simulink model "gm_uz_pmsm_model_6ph_dq"  (R2023a)
settings: Solver=FixedStepAuto  StartTime=0.0  StopTime=0.8  RelTol=1e-3
undefined symbols (not defined in the file or in its folder): c, friction_coefficient, inertia, k_i_d, k_i_q, k_p_d, k_p_q, Kpd, L_d, L_q, L_x, L_y, L_z1, L_z2, polepair, psi_pm, R_1, static_friction_torque, Tnd
libraries: hdlmdlgenlib x51, slpidlib x2, pid_lib x1, spsdq0toAlphaBetaZeroLib x1
(part 2 of 2)

== system gm_uz_pmsm_model_6ph_dq/uz_pmsm_model_6ph_dq/Data Type Conversion14 ==
  In1 : Inport
  Data Type Conversion14 : DataTypeConversion  OutDataTypeStr=single  RndMeth=Nearest  SampleTime=1e-08  SaturateOnIntegerOverflow=off
  Data Type Conversion14_pd1 : Delay  DelayLength=3
  Out1 : Outport
  wires:
  In1/1 -> Data Type Conversion14/1
  Data Type Conversion14/1 -> Data Type Conversion14_pd1/1
  Data Type Conversion14_pd1/1 -> Out1/1

== system gm_uz_pmsm_model_6ph_dq/uz_pmsm_model_6ph_dq/Data Type Conversion15 ==
  In1 : Inport
  Data Type Conversion15 : DataTypeConversion  OutDataTypeStr=double  RndMeth=Nearest  SampleTime=1e-08  SaturateOnIntegerOverflow=off
  Data Type Conversion15_pd1 : Delay  DelayLength=3
  Out1 : Outport
  wires:
  In1/1 -> Data Type Conversion15/1
  Data Type Conversion15/1 -> Data Type Conversion15_pd1/1
  Data Type Conversion15_pd1/1 -> Out1/1

== system gm_uz_pmsm_model_6ph_dq/uz_pmsm_model_6ph_dq/Data Type Conversion2 ==
  In1 : Inport
  Data Type Conversion2 : DataTypeConversion  OutDataTypeStr=double  RndMeth=Nearest  SampleTime=1e-08  SaturateOnIntegerOverflow=off
  Data Type Conversion2_pd1 : Delay  DelayLength=3
  Out1 : Outport
  wires:
  In1/1 -> Data Type Conversion2/1
  Data Type Conversion2/1 -> Data Type Conversion2_pd1/1
  Data Type Conversion2_pd1/1 -> Out1/1

== system gm_uz_pmsm_model_6ph_dq/uz_pmsm_model_6ph_dq/Data Type Conversion21 ==
  In1 : Inport
  Data Type Conversion21 : DataTypeConversion  OutDataTypeStr=double  RndMeth=Nearest  SampleTime=1e-08  SaturateOnIntegerOverflow=off
  Data Type Conversion21_pd1 : Delay  DelayLength=3
  Out1 : Outport
  wires:
  In1/1 -> Data Type Conversion21/1
  Data Type Conversion21/1 -> Data Type Conversion21_pd1/1
  Data Type Conversion21_pd1/1 -> Out1/1

== system gm_uz_pmsm_model_6ph_dq/uz_pmsm_model_6ph_dq/Data Type Conversion3 ==
  In1 : Inport
  Data Type Conversion3 : DataTypeConversion  OutDataTypeStr=fixdt(1, 27, 18)  RndMeth=Nearest  SampleTime=1e-08  SaturateOnIntegerOverflow=off
  Data Type Conversion3_pd1 : Delay  DelayLength=3
  Out1 : Outport
  wires:
  In1/1 -> Data Type Conversion3/1
  Data Type Conversion3/1 -> Data Type Conversion3_pd1/1
  Data Type Conversion3_pd1/1 -> Out1/1

== system gm_uz_pmsm_model_6ph_dq/uz_pmsm_model_6ph_dq/Data Type Conversion31 ==
  In1 : Inport
  Data Type Conversion31 : DataTypeConversion  OutDataTypeStr=double  RndMeth=Nearest  SampleTime=1e-08  SaturateOnIntegerOverflow=off
  Data Type Conversion31_pd1 : Delay  DelayLength=3
  Out1 : Outport
  wires:
  In1/1 -> Data Type Conversion31/1
  Data Type Conversion31/1 -> Data Type Conversion31_pd1/1
  Data Type Conversion31_pd1/1 -> Out1/1

== system gm_uz_pmsm_model_6ph_dq/uz_pmsm_model_6ph_dq/Data Type Conversion4 ==
  In1 : Inport
  Data Type Conversion4 : DataTypeConversion  OutDataTypeStr=single  RndMeth=Nearest  SampleTime=1e-08  SaturateOnIntegerOverflow=off
  Data Type Conversion4_pd1 : Delay  DelayLength=3
  Out1 : Outport
  wires:
  In1/1 -> Data Type Conversion4/1
  Data Type Conversion4/1 -> Data Type Conversion4_pd1/1
  Data Type Conversion4_pd1/1 -> Out1/1

== system gm_uz_pmsm_model_6ph_dq/uz_pmsm_model_6ph_dq/Data Type Conversion41 ==
  In1 : Inport
  Data Type Conversion41 : DataTypeConversion  OutDataTypeStr=double  RndMeth=Nearest  SampleTime=1e-08  SaturateOnIntegerOverflow=off
  Data Type Conversion41_pd1 : Delay  DelayLength=3
  Out1 : Outport
  wires:
  In1/1 -> Data Type Conversion41/1
  Data Type Conversion41/1 -> Data Type Conversion41_pd1/1
  Data Type Conversion41_pd1/1 -> Out1/1

== system gm_uz_pmsm_model_6ph_dq/uz_pmsm_model_6ph_dq/Data Type Conversion5 ==
  In1 : Inport
  Data Type Conversion5 : DataTypeConversion  OutDataTypeStr=single  RndMeth=Nearest  SampleTime=1e-08  SaturateOnIntegerOverflow=off
  Data Type Conversion5_pd1 : Delay  DelayLength=3
  Out1 : Outport
  wires:
  In1/1 -> Data Type Conversion5/1
  Data Type Conversion5/1 -> Data Type Conversion5_pd1/1
  Data Type Conversion5_pd1/1 -> Out1/1

== system gm_uz_pmsm_model_6ph_dq/uz_pmsm_model_6ph_dq/Data Type Conversion51 ==
  In1 : Inport
  Data Type Conversion51 : DataTypeConversion  OutDataTypeStr=double  RndMeth=Nearest  SampleTime=1e-08  SaturateOnIntegerOverflow=off
  Data Type Conversion51_pd1 : Delay  DelayLength=3
  Out1 : Outport
  wires:
  In1/1 -> Data Type Conversion51/1
  Data Type Conversion51/1 -> Data Type Conversion51_pd1/1
  Data Type Conversion51_pd1/1 -> Out1/1

== system gm_uz_pmsm_model_6ph_dq/uz_pmsm_model_6ph_dq/Data Type Conversion6 ==
  In1 : Inport
  Data Type Conversion6 : DataTypeConversion  OutDataTypeStr=double  RndMeth=Nearest  SampleTime=1e-08  SaturateOnIntegerOverflow=off
  Data Type Conversion6_pd1 : Delay  DelayLength=3
  Out1 : Outport
  wires:
  In1/1 -> Data Type Conversion6/1
  Data Type Conversion6/1 -> Data Type Conversion6_pd1/1
  Data Type Conversion6_pd1/1 -> Out1/1

== system gm_uz_pmsm_model_6ph_dq/uz_pmsm_model_6ph_dq/Data Type Conversion61 ==
  In1 : Inport
  Data Type Conversion61 : DataTypeConversion  OutDataTypeStr=double  RndMeth=Nearest  SampleTime=1e-08  SaturateOnIntegerOverflow=off
  Data Type Conversion61_pd1 : Delay  DelayLength=3
  Out1 : Outport
  wires:
  In1/1 -> Data Type Conversion61/1
  Data Type Conversion61/1 -> Data Type Conversion61_pd1/1
  Data Type Conversion61_pd1/1 -> Out1/1

== system gm_uz_pmsm_model_6ph_dq/uz_pmsm_model_6ph_dq/Data Type Conversion7 ==
  In1 : Inport
  Data Type Conversion7 : DataTypeConversion  OutDataTypeStr=double  RndMeth=Nearest  SampleTime=1e-08  SaturateOnIntegerOverflow=off
  Data Type Conversion7_pd1 : Delay  DelayLength=3
  Out1 : Outport
  wires:
  In1/1 -> Data Type Conversion7/1
  Data Type Conversion7/1 -> Data Type Conversion7_pd1/1
  Data Type Conversion7_pd1/1 -> Out1/1

== system gm_uz_pmsm_model_6ph_dq/uz_pmsm_model_6ph_dq/Data Type Conversion71 ==
  In1 : Inport
  Data Type Conversion71 : DataTypeConversion  OutDataTypeStr=double  RndMeth=Nearest  SampleTime=1e-08  SaturateOnIntegerOverflow=off
  Data Type Conversion71_pd1 : Delay  DelayLength=3
  Out1 : Outport
  wires:
  In1/1 -> Data Type Conversion71/1
  Data Type Conversion71/1 -> Data Type Conversion71_pd1/1
  Data Type Conversion71_pd1/1 -> Out1/1

== system gm_uz_pmsm_model_6ph_dq/uz_pmsm_model_6ph_dq/Data Type Conversion8 ==
  In1 : Inport
  Data Type Conversion8 : DataTypeConversion  OutDataTypeStr=double  RndMeth=Nearest  SampleTime=1e-08  SaturateOnIntegerOverflow=off
  Data Type Conversion8_pd1 : Delay  DelayLength=3
  Out1 : Outport
  wires:
  In1/1 -> Data Type Conversion8/1
  Data Type Conversion8/1 -> Data Type Conversion8_pd1/1
  Data Type Conversion8_pd1/1 -> Out1/1

== system gm_uz_pmsm_model_6ph_dq/uz_pmsm_model_6ph_dq/Data Type Conversion81 ==
  In1 : Inport
  Data Type Conversion81 : DataTypeConversion  OutDataTypeStr=single  RndMeth=Nearest  SampleTime=1e-08  SaturateOnIntegerOverflow=off
  Data Type Conversion81_pd1 : Delay  DelayLength=3
  Out1 : Outport
  wires:
  In1/1 -> Data Type Conversion81/1
  Data Type Conversion81/1 -> Data Type Conversion81_pd1/1
  Data Type Conversion81_pd1/1 -> Out1/1

== system gm_uz_pmsm_model_6ph_dq/uz_pmsm_model_6ph_dq/Data Type Conversion9 ==
  In1 : Inport
  Data Type Conversion9 : DataTypeConversion  OutDataTypeStr=fixdt(1, 24, 11)  RndMeth=Nearest  SampleTime=1e-08  SaturateOnIntegerOverflow=off
  Data Type Conversion9_pd1 : Delay  DelayLength=6
  Out1 : Outport
  wires:
  In1/1 -> Data Type Conversion9/1
  Data Type Conversion9/1 -> Data Type Conversion9_pd1/1
  Data Type Conversion9_pd1/1 -> Out1/1

== system gm_uz_pmsm_model_6ph_dq/uz_pmsm_model_6ph_dq/Data Type Conversion91 ==
  In1 : Inport
  Data Type Conversion91 : DataTypeConversion  OutDataTypeStr=double  RndMeth=Nearest  SampleTime=1e-08  SaturateOnIntegerOverflow=off
  Data Type Conversion91_pd1 : Delay  DelayLength=3
  Out1 : Outport
  wires:
  In1/1 -> Data Type Conversion91/1
  Data Type Conversion91/1 -> Data Type Conversion91_pd1/1
  Data Type Conversion91_pd1/1 -> Out1/1

== system gm_uz_pmsm_model_6ph_dq/uz_pmsm_model_6ph_dq/Divide ==
  In1 : Inport
  In2 : Inport  Port=2
  Divide : Product  Inputs=**  OutDataTypeStr=double  SampleTime=1e-08
  Divide_pd1 : Delay  DelayLength=6
  Out1 : Outport
  wires:
  In1/1 -> Divide/1
  In2/1 -> Divide/2
  Divide/1 -> Divide_pd1/1
  Divide_pd1/1 -> Out1/1

== system gm_uz_pmsm_model_6ph_dq/uz_pmsm_model_6ph_dq/Divide1 ==
  In1 : Inport
  In2 : Inport  Port=2
  Divide1 : Product  Inputs=**  OutDataTypeStr=double  SampleTime=1e-08
  Divide1_pd1 : Delay  DelayLength=6
  Out1 : Outport
  wires:
  In1/1 -> Divide1/1
  In2/1 -> Divide1/2
  Divide1/1 -> Divide1_pd1/1
  Divide1_pd1/1 -> Out1/1

== system gm_uz_pmsm_model_6ph_dq/uz_pmsm_model_6ph_dq/Divide11 ==
  In1 : Inport
  In2 : Inport  Port=2
  Divide11 : Product  Inputs=**  OutDataTypeStr=double  SampleTime=1e-08
  Divide11_pd1 : Delay  DelayLength=6
  Out1 : Outport
  wires:
  In1/1 -> Divide11/1
  In2/1 -> Divide11/2
  Divide11/1 -> Divide11_pd1/1
  Divide11_pd1/1 -> Out1/1

== system gm_uz_pmsm_model_6ph_dq/uz_pmsm_model_6ph_dq/Divide2 ==
  In1 : Inport
  In2 : Inport  Port=2
  Divide2 : Product  Inputs=**  OutDataTypeStr=double  SampleTime=1e-08
  Divide2_pd1 : Delay  DelayLength=6
  Out1 : Outport
  wires:
  In1/1 -> Divide2/1
  In2/1 -> Divide2/2
  Divide2/1 -> Divide2_pd1/1
  Divide2_pd1/1 -> Out1/1

== system gm_uz_pmsm_model_6ph_dq/uz_pmsm_model_6ph_dq/Divide3 ==
  In1 : Inport
  In2 : Inport  Port=2
  Divide3 : Product  Inputs=**  OutDataTypeStr=double  SampleTime=1e-08
  Divide3_pd1 : Delay  DelayLength=6
  Out1 : Outport
  wires:
  In1/1 -> Divide3/1
  In2/1 -> Divide3/2
  Divide3/1 -> Divide3_pd1/1
  Divide3_pd1/1 -> Out1/1

== system gm_uz_pmsm_model_6ph_dq/uz_pmsm_model_6ph_dq/Divide4 ==
  In1 : Inport
  In2 : Inport  Port=2
  Divide4 : Product  Inputs=**  OutDataTypeStr=double  SampleTime=1e-08
  Divide4_pd1 : Delay  DelayLength=6
  Out1 : Outport
  wires:
  In1/1 -> Divide4/1
  In2/1 -> Divide4/2
  Divide4/1 -> Divide4_pd1/1
  Divide4_pd1/1 -> Out1/1

== system gm_uz_pmsm_model_6ph_dq/uz_pmsm_model_6ph_dq/Divide5 ==
  In1 : Inport
  In2 : Inport  Port=2
  Divide5 : Product  Inputs=**  OutDataTypeStr=double  SampleTime=1e-08
  Divide5_pd1 : Delay  DelayLength=6
  Out1 : Outport
  wires:
  In1/1 -> Divide5/1
  In2/1 -> Divide5/2
  Divide5/1 -> Divide5_pd1/1
  Divide5_pd1/1 -> Out1/1

== system gm_uz_pmsm_model_6ph_dq/uz_pmsm_model_6ph_dq/Divide6 ==
  In1 : Inport
  In2 : Inport  Port=2
  Divide6 : Product  Inputs=**  OutDataTypeStr=double  SampleTime=1e-08
  Divide6_pd1 : Delay  DelayLength=6
  Out1 : Outport
  wires:
  In1/1 -> Divide6/1
  In2/1 -> Divide6/2
  Divide6/1 -> Divide6_pd1/1
  Divide6_pd1/1 -> Out1/1

== system gm_uz_pmsm_model_6ph_dq/uz_pmsm_model_6ph_dq/Divide7 ==
  In1 : Inport
  In2 : Inport  Port=2
  Divide7 : Product  Inputs=**  OutDataTypeStr=double  SampleTime=1e-08
  Divide7_pd1 : Delay  DelayLength=6
  Out1 : Outport
  wires:
  In1/1 -> Divide7/1
  In2/1 -> Divide7/2
  Divide7/1 -> Divide7_pd1/1
  Divide7_pd1/1 -> Out1/1

== system gm_uz_pmsm_model_6ph_dq/uz_pmsm_model_6ph_dq/Divide9 ==
  In1 : Inport
  In2 : Inport  Port=2
  Divide9 : Product  Inputs=**  OutDataTypeStr=double  SampleTime=1e-08
  Divide9_pd1 : Delay  DelayLength=6
  Out1 : Outport
  wires:
  In1/1 -> Divide9/1
  In2/1 -> Divide9/2
  Divide9/1 -> Divide9_pd1/1
  Divide9_pd1/1 -> Out1/1

== system gm_uz_pmsm_model_6ph_dq/uz_pmsm_model_6ph_dq/Factor ==
  In1 : Inport
  In2 : Inport  Port=2
  Factor : Product  Inputs=**  OutDataTypeStr=double  SampleTime=1e-08
  Factor_pd1 : Delay  DelayLength=6
  Out1 : Outport
  wires:
  In1/1 -> Factor/1
  In2/1 -> Factor/2
  Factor/1 -> Factor_pd1/1
  Factor_pd1/1 -> Out1/1

== system gm_uz_pmsm_model_6ph_dq/uz_pmsm_model_6ph_dq/Gain ==
  In1 : Inport
  In2 : Inport  Port=2
  Gain : Product  Inputs=**  OutDataTypeStr=double  SampleTime=1e-08
  Gain_pd1 : Delay  DelayLength=6
  Out1 : Outport
  wires:
  In1/1 -> Gain/1
  In2/1 -> Gain/2
  Gain/1 -> Gain_pd1/1
  Gain_pd1/1 -> Out1/1

== system gm_uz_pmsm_model_6ph_dq/uz_pmsm_model_6ph_dq/Gain1 ==
  In1 : Inport
  In2 : Inport  Port=2
  Gain1 : Product  Inputs=**  OutDataTypeStr=double  SampleTime=1e-08
  Gain1_pd1 : Delay  DelayLength=6
  Out1 : Outport
  wires:
  In1/1 -> Gain1/1
  In2/1 -> Gain1/2
  Gain1/1 -> Gain1_pd1/1
  Gain1_pd1/1 -> Out1/1

== system gm_uz_pmsm_model_6ph_dq/uz_pmsm_model_6ph_dq/Gain2 ==
  In1 : Inport
  In2 : Inport  Port=2
  Gain2 : Product  Inputs=**  OutDataTypeStr=double  SampleTime=1e-08
  Gain2_pd1 : Delay  DelayLength=6
  Out1 : Outport
  wires:
  In1/1 -> Gain2/1
  In2/1 -> Gain2/2
  Gain2/1 -> Gain2_pd1/1
  Gain2_pd1/1 -> Out1/1

== system gm_uz_pmsm_model_6ph_dq/uz_pmsm_model_6ph_dq/Gain3 ==
  In1 : Inport
  In2 : Inport  Port=2
  Gain3 : Product  Inputs=**  OutDataTypeStr=double  SampleTime=1e-08
  Gain3_pd1 : Delay  DelayLength=6
  Out1 : Outport
  wires:
  In1/1 -> Gain3/1
  In2/1 -> Gain3/2
  Gain3/1 -> Gain3_pd1/1
  Gain3_pd1/1 -> Out1/1

== system gm_uz_pmsm_model_6ph_dq/uz_pmsm_model_6ph_dq/Gain4 ==
  In1 : Inport
  In2 : Inport  Port=2
  Gain4 : Product  Inputs=**  OutDataTypeStr=double  SampleTime=1e-08
  Gain4_pd1 : Delay  DelayLength=6
  Out1 : Outport
  wires:
  In1/1 -> Gain4/1
  In2/1 -> Gain4/2
  Gain4/1 -> Gain4_pd1/1
  Gain4_pd1/1 -> Out1/1

== system gm_uz_pmsm_model_6ph_dq/uz_pmsm_model_6ph_dq/Gain5 ==
  In1 : Inport
  In2 : Inport  Port=2
  Gain5 : Product  Inputs=**  OutDataTypeStr=double  SampleTime=1e-08
  Gain5_pd1 : Delay  DelayLength=6
  Out1 : Outport
  wires:
  In1/1 -> Gain5/1
  In2/1 -> Gain5/2
  Gain5/1 -> Gain5_pd1/1
  Gain5_pd1/1 -> Out1/1

== system gm_uz_pmsm_model_6ph_dq/uz_pmsm_model_6ph_dq/Gain6 ==
  In1 : Inport
  In2 : Inport  Port=2
  Gain6 : Product  Inputs=**  OutDataTypeStr=double  SampleTime=1e-08
  Gain6_pd1 : Delay  DelayLength=6
  Out1 : Outport
  wires:
  In1/1 -> Gain6/1
  In2/1 -> Gain6/2
  Gain6/1 -> Gain6_pd1/1
  Gain6_pd1/1 -> Out1/1

== system gm_uz_pmsm_model_6ph_dq/uz_pmsm_model_6ph_dq/Gain7 ==
  In1 : Inport
  In2 : Inport  Port=2
  Gain7 : Product  Inputs=**  OutDataTypeStr=double  SampleTime=1e-08
  Gain7_pd1 : Delay  DelayLength=6
  Out1 : Outport
  wires:
  In1/1 -> Gain7/1
  In2/1 -> Gain7/2
  Gain7/1 -> Gain7_pd1/1
  Gain7_pd1/1 -> Out1/1

== system gm_uz_pmsm_model_6ph_dq/uz_pmsm_model_6ph_dq/Product ==
  In1 : Inport
  In2 : Inport  Port=2
  Product : Product  Inputs=**  OutDataTypeStr=double  SampleTime=1e-08
  Product_pd1 : Delay  DelayLength=6
  Out1 : Outport
  wires:
  In1/1 -> Product/1
  In2/1 -> Product/2
  Product/1 -> Product_pd1/1
  Product_pd1/1 -> Out1/1

== system gm_uz_pmsm_model_6ph_dq/uz_pmsm_model_6ph_dq/Product1 ==
  In1 : Inport
  In2 : Inport  Port=2
  Product1 : Product  Inputs=**  OutDataTypeStr=double  SampleTime=1e-08
  Product1_pd1 : Delay  DelayLength=6
  Out1 : Outport
  wires:
  In1/1 -> Product1/1
  In2/1 -> Product1/2
  Product1/1 -> Product1_pd1/1
  Product1_pd1/1 -> Out1/1

== system gm_uz_pmsm_model_6ph_dq/uz_pmsm_model_6ph_dq/Product10 ==
  In1 : Inport
  In2 : Inport  Port=2
  Product10 : Product  Inputs=**  OutDataTypeStr=double  SampleTime=1e-08
  Product10_pd1 : Delay  DelayLength=6
  Out1 : Outport
  wires:
  In1/1 -> Product10/1
  In2/1 -> Product10/2
  Product10/1 -> Product10_pd1/1
  Product10_pd1/1 -> Out1/1

== system gm_uz_pmsm_model_6ph_dq/uz_pmsm_model_6ph_dq/Product11 ==
  In1 : Inport
  In2 : Inport  Port=2
  Product11 : Product  Inputs=**  OutDataTypeStr=double  SampleTime=1e-08
  Product11_pd1 : Delay  DelayLength=6
  Out1 : Outport
  wires:
  In1/1 -> Product11/1
  In2/1 -> Product11/2
  Product11/1 -> Product11_pd1/1
  Product11_pd1/1 -> Out1/1

== system gm_uz_pmsm_model_6ph_dq/uz_pmsm_model_6ph_dq/Product2 ==
  In1 : Inport
  In2 : Inport  Port=2
  Product2 : Product  Inputs=**  OutDataTypeStr=double  SampleTime=1e-08
  Product2_pd1 : Delay  DelayLength=6
  Out1 : Outport
  wires:
  In1/1 -> Product2/1
  In2/1 -> Product2/2
  Product2/1 -> Product2_pd1/1
  Product2_pd1/1 -> Out1/1

== system gm_uz_pmsm_model_6ph_dq/uz_pmsm_model_6ph_dq/Product21 ==
  In1 : Inport
  In2 : Inport  Port=2
  Product21 : Product  Inputs=**  OutDataTypeStr=double  SampleTime=1e-08
  Product21_pd1 : Delay  DelayLength=6
  Out1 : Outport
  wires:
  In1/1 -> Product21/1
  In2/1 -> Product21/2
  Product21/1 -> Product21_pd1/1
  Product21_pd1/1 -> Out1/1

== system gm_uz_pmsm_model_6ph_dq/uz_pmsm_model_6ph_dq/Product3 ==
  In1 : Inport
  In2 : Inport  Port=2
  Product3 : Product  Inputs=**  OutDataTypeStr=double  SampleTime=1e-08
  Product3_pd1 : Delay  DelayLength=6
  Out1 : Outport
  wires:
  In1/1 -> Product3/1
  In2/1 -> Product3/2
  Product3/1 -> Product3_pd1/1
  Product3_pd1/1 -> Out1/1

== system gm_uz_pmsm_model_6ph_dq/uz_pmsm_model_6ph_dq/Product5 ==
  In1 : Inport
  In2 : Inport  Port=2
  Product5 : Product  Inputs=**  OutDataTypeStr=double  SampleTime=1e-08
  Product5_pd1 : Delay  DelayLength=6
  Out1 : Outport
  wires:
  In1/1 -> Product5/1
  In2/1 -> Product5/2
  Product5/1 -> Product5_pd1/1
  Product5_pd1/1 -> Out1/1

== system gm_uz_pmsm_model_6ph_dq/uz_pmsm_model_6ph_dq/Product6 ==
  In1 : Inport
  In2 : Inport  Port=2
  Product6 : Product  Inputs=**  OutDataTypeStr=double  SampleTime=1e-08
  Product6_pd1 : Delay  DelayLength=6
  Out1 : Outport
  wires:
  In1/1 -> Product6/1
  In2/1 -> Product6/2
  Product6/1 -> Product6_pd1/1
  Product6_pd1/1 -> Out1/1

== system gm_uz_pmsm_model_6ph_dq/uz_pmsm_model_6ph_dq/Product7 ==
  In1 : Inport
  In2 : Inport  Port=2
  Product7 : Product  Inputs=**  OutDataTypeStr=double  SampleTime=1e-08
  Product7_pd1 : Delay  DelayLength=6
  Out1 : Outport
  wires:
  In1/1 -> Product7/1
  In2/1 -> Product7/2
  Product7/1 -> Product7_pd1/1
  Product7_pd1/1 -> Out1/1

== system gm_uz_pmsm_model_6ph_dq/uz_pmsm_model_6ph_dq/Product8 ==
  In1 : Inport
  In2 : Inport  Port=2
  Product8 : Product  Inputs=**  OutDataTypeStr=double  SampleTime=1e-08
  Product8_pd1 : Delay  DelayLength=6
  Out1 : Outport
  wires:
  In1/1 -> Product8/1
  In2/1 -> Product8/2
  Product8/1 -> Product8_pd1/1
  Product8_pd1/1 -> Out1/1

== system gm_uz_pmsm_model_6ph_dq/uz_pmsm_model_6ph_dq/Product9 ==
  In1 : Inport
  In2 : Inport  Port=2
  Product9 : Product  Inputs=**  OutDataTypeStr=double  SampleTime=1e-08
  Product9_pd1 : Delay  DelayLength=6
  Out1 : Outport
  wires:
  In1/1 -> Product9/1
  In2/1 -> Product9/2
  Product9/1 -> Product9_pd1/1
  Product9_pd1/1 -> Out1/1

== system gm_uz_pmsm_model_6ph_dq/uz_pmsm_model_6ph_dq/Sum ==
  In1 : Inport
  In2 : Inport  Port=2
  Sum : Sum  OutDataTypeStr=double  SampleTime=1e-08
  Sum_pd1 : Delay  DelayLength=6
  Out1 : Outport
  wires:
  In1/1 -> Sum/1
  In2/1 -> Sum/2
  Sum/1 -> Sum_pd1/1
  Sum_pd1/1 -> Out1/1

== system gm_uz_pmsm_model_6ph_dq/uz_pmsm_model_6ph_dq/Sum1 ==
  In1 : Inport
  In2 : Inport  Port=2
  Sum1 : Sum  OutDataTypeStr=double  SampleTime=1e-08
  Sum1_pd1 : Delay  DelayLength=6
  Out1 : Outport
  wires:
  In1/1 -> Sum1/1
  In2/1 -> Sum1/2
  Sum1/1 -> Sum1_pd1/1
  Sum1_pd1/1 -> Out1/1

== system gm_uz_pmsm_model_6ph_dq/uz_pmsm_model_6ph_dq/Sum11 ==
  In1 : Inport
  In2 : Inport  Port=2
  Sum11 : Sum  Inputs=+-  OutDataTypeStr=double  SampleTime=1e-08
  Sum11_pd1 : Delay  DelayLength=6
  Out1 : Outport
  wires:
  In1/1 -> Sum11/1
  In2/1 -> Sum11/2
  Sum11/1 -> Sum11_pd1/1
  Sum11_pd1/1 -> Out1/1

== system gm_uz_pmsm_model_6ph_dq/uz_pmsm_model_6ph_dq/Sum1_stage2 ==
  In1 : Inport
  In2 : Inport  Port=2
  Sum1_stage2 : Sum  Inputs=+-  OutDataTypeStr=double  SampleTime=1e-08
  Sum1_stage2_pd1 : Delay  DelayLength=6
  Out1 : Outport
  wires:
  In1/1 -> Sum1_stage2/1
  In2/1 -> Sum1_stage2/2
  Sum1_stage2/1 -> Sum1_stage2_pd1/1
  Sum1_stage2_pd1/1 -> Out1/1

== system gm_uz_pmsm_model_6ph_dq/uz_pmsm_model_6ph_dq/Sum1_stage3 ==
  In1 : Inport
  In2 : Inport  Port=2
  Sum1_stage3 : Sum  Inputs=+-  OutDataTypeStr=double  SampleTime=1e-08
  Sum1_stage3_pd1 : Delay  DelayLength=6
  Out1 : Outport
  wires:
  In1/1 -> Sum1_stage3/1
  In2/1 -> Sum1_stage3/2
  Sum1_stage3/1 -> Sum1_stage3_pd1/1
  Sum1_stage3_pd1/1 -> Out1/1

== system gm_uz_pmsm_model_6ph_dq/uz_pmsm_model_6ph_dq/Sum2 ==
  In1 : Inport
  In2 : Inport  Port=2
  Sum2 : Sum  OutDataTypeStr=double  SampleTime=1e-08
  Sum2_pd1 : Delay  DelayLength=6
  Out1 : Outport
  wires:
  In1/1 -> Sum2/1
  In2/1 -> Sum2/2
  Sum2/1 -> Sum2_pd1/1
  Sum2_pd1/1 -> Out1/1

== system gm_uz_pmsm_model_6ph_dq/uz_pmsm_model_6ph_dq/Sum21 ==
  In1 : Inport
  In2 : Inport  Port=2
  Sum21 : Sum  Inputs=+-  OutDataTypeStr=double  SampleTime=1e-08
  Sum21_pd1 : Delay  DelayLength=6
  Out1 : Outport
  wires:
  In1/1 -> Sum21/1
  In2/1 -> Sum21/2
  Sum21/1 -> Sum21_pd1/1
  Sum21_pd1/1 -> Out1/1

== system gm_uz_pmsm_model_6ph_dq/uz_pmsm_model_6ph_dq/Sum3 ==
  In1 : Inport
  In2 : Inport  Port=2
  Sum3 : Sum  OutDataTypeStr=double  SampleTime=1e-08
  Sum3_pd1 : Delay  DelayLength=6
  Out1 : Outport
  wires:
  In1/1 -> Sum3/1
  In2/1 -> Sum3/2
  Sum3/1 -> Sum3_pd1/1
  Sum3_pd1/1 -> Out1/1

== system gm_uz_pmsm_model_6ph_dq/uz_pmsm_model_6ph_dq/Sum31 ==
  In1 : Inport
  In2 : Inport  Port=2
  Sum31 : Sum  OutDataTypeStr=double  SampleTime=1e-08
  Sum31_pd1 : Delay  DelayLength=6
  Out1 : Outport
  wires:
  In1/1 -> Sum31/1
  In2/1 -> Sum31/2
  Sum31/1 -> Sum31_pd1/1
  Sum31_pd1/1 -> Out1/1

== system gm_uz_pmsm_model_6ph_dq/uz_pmsm_model_6ph_dq/Sum32 ==
  In1 : Inport
  In2 : Inport  Port=2
  Sum32 : Sum  OutDataTypeStr=double  SampleTime=1e-08
  Sum32_pd1 : Delay  DelayLength=6
  Out1 : Outport
  wires:
  In1/1 -> Sum32/1
  In2/1 -> Sum32/2
  Sum32/1 -> Sum32_pd1/1
  Sum32_pd1/1 -> Out1/1

== system gm_uz_pmsm_model_6ph_dq/uz_pmsm_model_6ph_dq/Sum33 ==
  In1 : Inport
  In2 : Inport  Port=2
  Sum33 : Sum  OutDataTypeStr=double  SampleTime=1e-08
  Sum33_pd1 : Delay  DelayLength=6
  Out1 : Outport
  wires:
  In1/1 -> Sum33/1
  In2/1 -> Sum33/2
  Sum33/1 -> Sum33_pd1/1
  Sum33_pd1/1 -> Out1/1

== system gm_uz_pmsm_model_6ph_dq/uz_pmsm_model_6ph_dq/Sum34 ==
  In1 : Inport
  In2 : Inport  Port=2
  Sum34 : Sum  OutDataTypeStr=double  SampleTime=1e-08
  Sum34_pd1 : Delay  DelayLength=6
  Out1 : Outport
  wires:
  In1/1 -> Sum34/1
  In2/1 -> Sum34/2
  Sum34/1 -> Sum34_pd1/1
  Sum34_pd1/1 -> Out1/1

== system gm_uz_pmsm_model_6ph_dq/uz_pmsm_model_6ph_dq/Sum35 ==
  In1 : Inport
  In2 : Inport  Port=2
  Sum35 : Sum  OutDataTypeStr=double  SampleTime=1e-08
  Sum35_pd1 : Delay  DelayLength=6
  Out1 : Outport
  wires:
  In1/1 -> Sum35/1
  In2/1 -> Sum35/2
  Sum35/1 -> Sum35_pd1/1
  Sum35_pd1/1 -> Out1/1

== system gm_uz_pmsm_model_6ph_dq/uz_pmsm_model_6ph_dq/Sum36 ==
  In1 : Inport
  In2 : Inport  Port=2
  Sum36 : Sum  OutDataTypeStr=double  SampleTime=1e-08
  Sum36_pd1 : Delay  DelayLength=6
  Out1 : Outport
  wires:
  In1/1 -> Sum36/1
  In2/1 -> Sum36/2
  Sum36/1 -> Sum36_pd1/1
  Sum36_pd1/1 -> Out1/1

== system gm_uz_pmsm_model_6ph_dq/uz_pmsm_model_6ph_dq/Sum37 ==
  In1 : Inport
  In2 : Inport  Port=2
  Sum37 : Sum  Inputs=+-  OutDataTypeStr=double  SampleTime=1e-08
  Sum37_pd1 : Delay  DelayLength=6
  Out1 : Outport
  wires:
  In1/1 -> Sum37/1
  In2/1 -> Sum37/2
  Sum37/1 -> Sum37_pd1/1
  Sum37_pd1/1 -> Out1/1

== system gm_uz_pmsm_model_6ph_dq/uz_pmsm_model_6ph_dq/Sum_stage2 ==
  In1 : Inport
  In2 : Inport  Port=2
  Sum_stage2 : Sum  Inputs=+-  OutDataTypeStr=double  SampleTime=1e-08
  Sum_stage2_pd1 : Delay  DelayLength=6
  Out1 : Outport
  wires:
  In1/1 -> Sum_stage2/1
  In2/1 -> Sum_stage2/2
  Sum_stage2/1 -> Sum_stage2_pd1/1
  Sum_stage2_pd1/1 -> Out1/1

== system gm_uz_pmsm_model_6ph_dq/uz_pmsm_model_6ph_dq/Sum_stage3 ==
  In1 : Inport
  In2 : Inport  Port=2
  Sum_stage3 : Sum  OutDataTypeStr=double  SampleTime=1e-08
  Sum_stage3_pd1 : Delay  DelayLength=6
  Out1 : Outport
  wires:
  In1/1 -> Sum_stage3/1
  In2/1 -> Sum_stage3/2
  Sum_stage3/1 -> Sum_stage3_pd1/1
  Sum_stage3_pd1/1 -> Out1/1
